simulink model "lumlummotor"  (R2020a)
settings: Solver=VariableStepAuto  StartTime=0.0  StopTime=10  RelTol=1e-3
values from neighbouring files (symbols this model uses):
  A = [0 1 0 ... (first row only)    [Lumlum.m]    (also in d_heli_2d_lqr_i.m = [; lumdownload.m; starter.m = [ 0    1.0000         0         0         0         0       )
  B = [0 0;0 -729.92; 641.81 0;]    [Lumlum.m]    (also in d_heli_2d_lqr_i.m = [; lumdownload.m = [0 0; starter.m = [ 0         0)
  C = eye(3)    [Lumlum.m]    (also in d_heli_2d_lqr_i.m = [; lumdownload.m; starter.m = eye(7))
  D = zeros(3,2)    [Lumlum.m]    (also in d_heli_2d_lqr_i.m = zeros(6,2); lumdownload.m; starter.m = zeros(7,2))
  K = tf([B1 B0], [A1 A0])    [HelicopterHoverExample.m]    (also in Lumlum.m = place(A,B,desired_eigen); lumdownload.m = place(A,B(:,1),desired_closed_loop_poles))
settings Model: Creator=Khojasteh Mirza  LastModifiedBy=Khojasteh Mirza

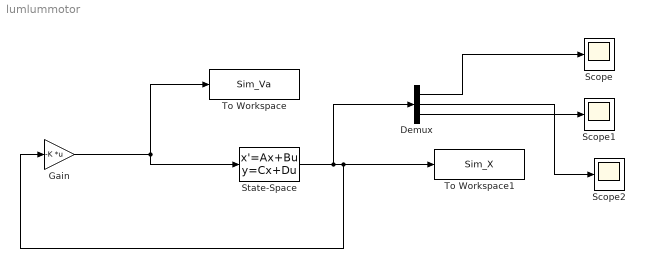
== system lumlummotor ==
  Demux : Demux  Outputs=3
  Gain : Gain  Gain=-K  Multiplication=Matrix(K*u)
  Scope : Scope
  Scope1 : Scope
  Scope2 : Scope
  State-Space : StateSpace  A=A  B=B  C=C  D=D  InitialCondition=[1;4;0]
  To Workspace : ToWorkspace  VariableName=Sim_Va  SaveFormat=Structure With Time  SampleTime=-1
  To Workspace1 : ToWorkspace  VariableName=Sim_X  SaveFormat=Structure With Time  SampleTime=-1
  wires:
  State-Space/1 -> Demux/1, To Workspace1/1, Gain/1
  Demux/1 -> Scope/1
  Demux/3 -> Scope1/1
  Demux/2 -> Scope2/1
  Gain/1 -> State-Space/1, To Workspace/1
